simulink model "TCMSSystem"  (R2019b)
settings: configuration reference "ConfigSet_TCMSSystem_Reference" (kept outside this file)
model workspace (MAT data in the model file):
  Prm_TCMSSystem = Simulink.Parameter
  Prm_TCMSSystem.Value.LoadCompensationMasses = [21000 33350]
  Prm_TCMSSystem.Value.LoadCompensationPressures = [165000 440000]
  Prm_TCMSSystem.Value.TractionAccelerationTargets = [0 1.36]
  Prm_TCMSSystem.Value.BrakingDecelerationTargets = [0 1.1]
  Prm_TCMSSystem.Value.TractionBrakingDemands = [0 100]
  Prm_TCMSSystem.Value.AW3TractionAccelerationTargets = [0 1.08]
  Prm_TCMSSystem.Value.AW3BrakingDecelerationTargets = [0 0.8]
  Prm_TCMSSystem.DataType = 'Bus: BD_TCMSSystem_Prm'
  Prm_TCMSSystem.Dimensions = [1 1]
  SampleTime = 0.05
undefined symbols (not defined in the file): ADDIntervention, AK1Status, AK2Status, AKContactorStatus, AllDoorsClosed, AllLeftDoorsClosed, AllRightDoorsClosed, APS1Fault, APS1Isolated, APS1OutputVoltage, APS1Status, APS2Fault, APS2Isolated, APS2OutputVoltage, APS2Status, APSKAKContactor, ASCOEnd1, ASCOEnd2, ATBMode, ATCBypassMode, ATCStatusNotOK, ATOMode, ATPLowSpeedCutoutStatus, ATPMode, AuxCompressor, BatteryCurrent, BatteryIsolationContactor, BatteryTemperature, BatteryVoltage, BCG1Fault, BCG1Isolated, BCG1IsolationFailed, BCG1OutputCurrent, BCG1Status, BCG2Fault, BCG2Isolated, BCG2OutputCurrent, BCG2Status, BCGOutputVoltage, BECU1AxleLockedWheelSet1, BECU2AxleLockedWheelSet2, BECUFaulty, BECUMajorFault, BECUMinorFault, BECUStatus, BIC1Inside, BIC1Outside, BIC2Inside, BIC2Outside, Bogie, Bogie1WSPStatus, Bogie2WSPStatus, BogieFaulty, BogieIsolationStatus, BogieSupportedMass, BrakeCylinderPressureGauge, BrakeLoopCBTripped, BrakeLoopOpenTL, BrakeTrainLineStatus, BrakingDemand ... (+215)
libraries: TimersLib x257, simulink x137, LatchesLib x42, VectorOperationsLib x15, TestBenchLib x12, MathOperationsLib x2, FiltersLib x1
(part 1 of 16)
settings Model: ParameterArgumentNames=Prm_TCMSSystem  Creator=cdyer  LastModifiedBy=hinganes
settings ConfigSetRef: SourceName=ConfigSet_TCMSSystem_Reference  SourceLocation=Base Workspace

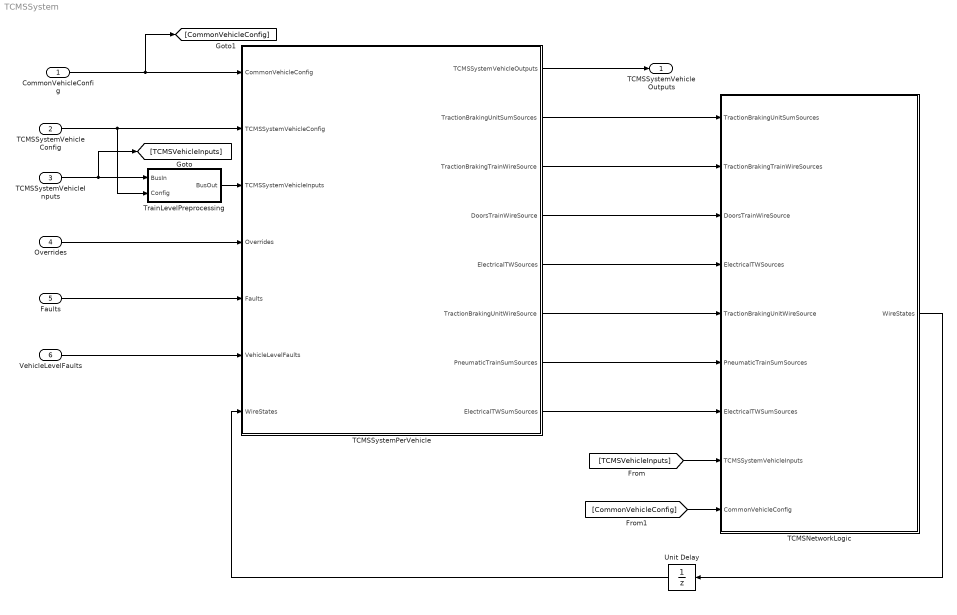
== system TCMSSystem ==
  CommonVehicleConfig : Inport  OutDataTypeStr=Bus: BD_CommonTrain_Cfg_Vehicle  PortDimensions=MaxVehicles  SampleTime=SampleTime  BusOutputAsStruct=on
  TCMSSystemVehicleConfig : Inport  Port=2  OutDataTypeStr=Bus: BD_TCMSSystem_Cfg_Vehicle  PortDimensions=MaxVehicles  SampleTime=SampleTime  BusOutputAsStruct=on
  TCMSSystemVehicleInputs : Inport  Port=3  OutDataTypeStr=Bus: BD_TCMSSystem_In_Vehicle  PortDimensions=MaxVehicles  SampleTime=SampleTime  BusOutputAsStruct=on
  Overrides : Inport  Port=4  OutDataTypeStr=Bus: BD_TCMSSystem_In_Vehicle_Overrides  PortDimensions=MaxVehicles  SampleTime=SampleTime  BusOutputAsStruct=on
  Faults : Inport  Port=5  OutDataTypeStr=Bus: BD_TCMSSystem_In_Vehicle_Faults  PortDimensions=MaxVehicles  SampleTime=SampleTime  BusOutputAsStruct=on
  VehicleLevelFaults : Inport  Port=6  OutDataTypeStr=Bus: BD_SimIntegration_Faults_Vehicle  PortDimensions=MaxVehicles  SampleTime=SampleTime  BusOutputAsStruct=on
  TCMSNetworkLogic : Subsystem  TreatAsAtomicUnit=on  SystemSampleTime=SampleTime
  TCMSSystemPerVehicle : Subsystem
  TrainLevelPreprocessing : Subsystem
  Unit Delay : UnitDelay  SampleTime=-1  HasFrameUpgradeWarning=on
  TCMSSystemVehicleOutputs : Outport  OutDataTypeStr=Bus: BD_TCMSSystem_Out_Vehicle  BusOutputAsStruct=on
  wires:
  CommonVehicleConfig/1 -> [CommonVehicleConfig], TCMSSystemPerVehicle/1(CommonVehicleConfig)
  TCMSSystemPerVehicle/1(TCMSSystemVehicleOutputs) -> TCMSSystemVehicleOutputs/1
  TCMSSystemVehicleConfig/1 -> TrainLevelPreprocessing/2(Config), TCMSSystemPerVehicle/2(TCMSSystemVehicleConfig)
  Overrides/1 -> TCMSSystemPerVehicle/4(Overrides)
  Faults/1 -> TCMSSystemPerVehicle/5(Faults)
  TCMSSystemPerVehicle/2(TractionBrakingUnitSumSources) -> TCMSNetworkLogic/1(TractionBrakingUnitSumSources)
  [TCMSVehicleInputs] -> TCMSNetworkLogic/8(TCMSSystemVehicleInputs)
  TCMSNetworkLogic/1(WireStates) -> Unit Delay/1
  Unit Delay/1 -> TCMSSystemPerVehicle/7(WireStates)
  TCMSSystemPerVehicle/3(TractionBrakingTrainWireSource) -> TCMSNetworkLogic/2(TractionBrakingTrainWireSources)
  TCMSSystemPerVehicle/4(DoorsTrainWireSource) -> TCMSNetworkLogic/3(DoorsTrainWireSource)
  TCMSSystemPerVehicle/5(ElectricalTWSources) -> TCMSNetworkLogic/4(ElectricalTWSources)
  [CommonVehicleConfig] -> TCMSNetworkLogic/9(CommonVehicleConfig)
  TCMSSystemPerVehicle/6(TractionBrakingUnitWireSource) -> TCMSNetworkLogic/5(TractionBrakingUnitWireSource)
  TCMSSystemPerVehicle/7(PneumaticTrainSumSources) -> TCMSNetworkLogic/6(PneumaticTrainSumSources)
  VehicleLevelFaults/1 -> TCMSSystemPerVehicle/6(VehicleLevelFaults)
  TCMSSystemPerVehicle/8(ElectricalTWSumSources) -> TCMSNetworkLogic/7(ElectricalTWSumSources)
  TCMSSystemVehicleInputs/1 -> [TCMSVehicleInputs], TrainLevelPreprocessing/1(BusIn)
  TrainLevelPreprocessing/1(BusOut) -> TCMSSystemPerVehicle/3(TCMSSystemVehicleInputs)

== system TCMSSystem/TCMSNetworkLogic ==
  TractionBrakingUnitSumSources : Inport  OutDataTypeStr=Bus: BD_TCMSSystem_Wires_TBUnitSum
  TractionBrakingTrainWireSources : Inport  Port=2  OutDataTypeStr=Bus: BD_TCMSSystem_Wires_TBTrainWire
  DoorsTrainWireSource : Inport  Port=3
  ElectricalTWSources : Inport  Port=4
  TractionBrakingUnitWireSource : Inport  Port=5
  PneumaticTrainSumSources : Inport  Port=6
  ElectricalTWSumSources : Inport  Port=7
  TCMSSystemVehicleInputs : Inport  Port=8  OutDataTypeStr=Bus: BD_TCMSSystem_In_Vehicle  PortDimensions=MaxVehicles  SampleTime=SampleTime  BusOutputAsStruct=on
  CommonVehicleConfig : Inport  Port=9
  ExtractConnections : Subsystem
  Goto Tag Visibility : GotoTagVisibility  GotoTag=Orientation
  Goto Tag Visibility1 : GotoTagVisibility  GotoTag=TrainConnection
  OrientationWiresLogic : Subsystem
  Terminator : Terminator
  TrainSumBus : VectorOperationsLib/TrainSumBus  OutDataTypeStr=Bus: BD_TCMSSystem_Wires_TBUnitSum
      settings: SourceProductName=Sydac Utilities
  TrainSumBus1 : VectorOperationsLib/TrainSumBus  OutDataTypeStr=Bus: BD_TCMSSystem_Wires_TBTrainWire
      settings: SourceProductName=Sydac Utilities
  TrainSumBus2 : VectorOperationsLib/TrainSumBus  OutDataTypeStr=Bus: BD_TCMSSystem_Wires_PneumaticTrainSum
      settings: SourceProductName=Sydac Utilities
  TrainSumBus3 : VectorOperationsLib/TrainSumBus  OutDataTypeStr=Bus: BD_TCMSSystem_Wires_ElectricalTrainSum
      settings: SourceProductName=Sydac Utilities
  TrainWiresBus : VectorOperationsLib/TrainWiresBus  OutDataTypeStr=Bus: BD_TCMSSystem_Wires_ElectricalTrainWire
      settings: SourceProductName=Sydac Utilities
  TrainWiresBus1 : VectorOperationsLib/TrainWiresBus  OutDataTypeStr=Bus: BD_TCMSSystem_Wires_TBUnitWire
      settings: SourceProductName=Sydac Utilities
  WireStatesRepack : Subsystem
  WireStates : Outport  OutDataTypeStr=Bus: BD_TCMSSystem_Wires
  tag scope: Orientation=scoped, TrainConnection=scoped
  wires:
  TractionBrakingUnitSumSources/1 -> TrainSumBus/1
  [UnitConnection] -> TrainSumBus/2
  TrainSumBus/1 -> WireStatesRepack/1(TractionBrakingUnitSumWireStates)
  TCMSSystemVehicleInputs/1 -> ExtractConnections/1(TCMSSystemVehicleInputs)
  ExtractConnections/1(UnitConnection) -> [UnitConnection]
  ExtractConnections/2(TrainConnection) -> [TrainConnection]
  [TrainConnection] -> TrainSumBus1/2
  TractionBrakingTrainWireSources/1 -> TrainSumBus1/1
  TrainSumBus1/1 -> WireStatesRepack/2(TractionBrakingTrainWireStates)
  WireStatesRepack/1(WireStates) -> WireStates/1
  ElectricalTWSources/1 -> TrainWiresBus/1
  [TrainConnection] -> TrainWiresBus/2
  TrainWiresBus/1 -> WireStatesRepack/4(ElectricalTrainWiresStates)
  CommonVehicleConfig/1 -> ExtractConnections/2(CommonVehicleConfig)
  ExtractConnections/3(Orientation) -> [Orientation]
  OrientationWiresLogic/1(WireStates) -> WireStatesRepack/3(DoorsTrainWiresStates)
  TractionBrakingUnitWireSource/1 -> TrainWiresBus1/1
  [UnitConnection] -> TrainWiresBus1/2
  TrainWiresBus1/1 -> WireStatesRepack/5(TractionBrakingUnitWire)
  TrainSumBus2/1 -> WireStatesRepack/6(PneumaticTrainSumSourcesWiresStates)
  PneumaticTrainSumSources/1 -> TrainSumBus2/1
  [TrainConnection] -> TrainSumBus2/2
  ElectricalTWSumSources/1 -> TrainSumBus3/1
  [TrainConnection] -> TrainSumBus3/2
  TrainSumBus3/1 -> WireStatesRepack/7(ElectricalTWSumSourcesWiresStates)
  [Orientation] -> Terminator/1
  DoorsTrainWireSource/1 -> OrientationWiresLogic/1(WireSources)

== system TCMSSystem/TCMSSystemPerVehicle ==
  CommonVehicleConfig : Inport  Partition=on  PartitionDimension=1  PartitionWidth=1  PartitionOffset=0
  TCMSSystemVehicleConfig : Inport  Port=2  Partition=on  PartitionDimension=1  PartitionWidth=1  PartitionOffset=0
  TCMSSystemVehicleInputs : Inport  Port=3  Partition=on  PartitionDimension=1  PartitionWidth=1  PartitionOffset=0
  Overrides : Inport  Port=4  Partition=on  PartitionDimension=1  PartitionWidth=1  PartitionOffset=0
  Faults : Inport  Port=5  Partition=on  PartitionDimension=1  PartitionWidth=1  PartitionOffset=0
  VehicleLevelFaults : Inport  Port=6  Partition=on  PartitionDimension=1  PartitionWidth=1  PartitionOffset=0
  WireStates : Inport  Port=7  Partition=on  PartitionDimension=1  PartitionWidth=1  PartitionOffset=0
  AND : Logic  AllPortsSameDT=off  OutDataTypeStr=boolean
  Bus Selector1 : BusSelector  OutputSignals=Enabled
  Bus Selector2 : BusSelector  OutputSignals=ElectricalSignals.TCMSPowerAvailable,ElectricalSignals.LimpHomeMode
  Bus Selector3 : BusSelector  OutputSignals=TCMSFailure
  Data Type Conversion : DataTypeConversion  OutDataTypeStr=uint32
  Data Type Conversion1 : DataTypeConversion  OutDataTypeStr=uint32
  Data Type Conversion2 : DataTypeConversion  OutDataTypeStr=uint32
  DisabledTCMSVehicle : Subsystem
  EnabledTCMSVehicle : Subsystem
  For Each : ForEach  DisableCoverage=on
  If : If  NumInputs=3  IfExpression=u1 > 0 & u2 ==0 & u3 == 1  ElseIfExpressions=u2 == 1
  LimpHomeTCMSVehicle : Subsystem
  Merge1 : Merge
  Merge3 : Merge
  Merge4 : Merge  Inputs=3
  Merge5 : Merge
  NOT : Logic  Operator=NOT  AllPortsSameDT=off  OutDataTypeStr=boolean
  Unit Delay : UnitDelay  SampleTime=-1  HasFrameUpgradeWarning=on
  TCMSSystemVehicleOutputs : Outport  ConcatenationDimension=1
  TractionBrakingUnitSumSources : Outport  Port=2  ConcatenationDimension=1
  TractionBrakingTrainWireSource : Outport  Port=3  ConcatenationDimension=1
  DoorsTrainWireSource : Outport  Port=4  ConcatenationDimension=1
  ElectricalTWSources : Outport  Port=5  ConcatenationDimension=1
  TractionBrakingUnitWireSource : Outport  Port=6  ConcatenationDimension=1
  PneumaticTrainSumSources : Outport  Port=7  ConcatenationDimension=1
  ElectricalTWSumSources : Outport  Port=8  ConcatenationDimension=1
  wires:
  CommonVehicleConfig/1 -> Bus Selector1/1, EnabledTCMSVehicle/1(CommonVehicleConfig)
  TCMSSystemVehicleConfig/1 -> DisabledTCMSVehicle/1(TCMSSystemVehicleConfig), LimpHomeTCMSVehicle/1(TCMSSystemVehicleConfig), EnabledTCMSVehicle/2(TCMSSystemVehicleConfig)
  Overrides/1 -> EnabledTCMSVehicle/4(Overrides)
  Faults/1 -> Bus Selector3/1, EnabledTCMSVehicle/5(TCMSFaults)
  Bus Selector2/1 -> AND/2  "<TCMSPowerAvailable>"
  Bus Selector1/1 -> AND/1  "<Enabled>"
  LimpHomeTCMSVehicle/3(NoTCMSSystemVehicleOutputs) -> Merge4/1
  If/2 -> LimpHomeTCMSVehicle/Action  "LimpHome"
  AND/1 -> Data Type Conversion/1
  If/1 -> EnabledTCMSVehicle/Action  "HealthyTCMS"
  Data Type Conversion/1 -> If/1
  EnabledTCMSVehicle/1(TractionBrakingUnitSumSources) -> Merge1/1
  WireStates/1 -> LimpHomeTCMSVehicle/3(WireStates), EnabledTCMSVehicle/6(WireStates)
  EnabledTCMSVehicle/2(TractionBrakingTrainWireSource) -> Merge5/1
  EnabledTCMSVehicle/4(DoorsTrainWireSource) -> DoorsTrainWireSource/1
  EnabledTCMSVehicle/3(ElectricalTWSources) -> ElectricalTWSources/1
  TCMSSystemVehicleInputs/1 -> Bus Selector2/1, LimpHomeTCMSVehicle/2(TCMSSystemInputs), EnabledTCMSVehicle/3(TCMSSystemInputs)
  Merge5/1 -> TractionBrakingTrainWireSource/1
  Merge1/1 -> TractionBrakingUnitSumSources/1
  LimpHomeTCMSVehicle/1(TractionBrakingUnitSumSources) -> Merge1/2
  LimpHomeTCMSVehicle/2(TractionBrakingTrainWireSource) -> Merge5/2
  Merge3/1 -> TractionBrakingUnitWireSource/1
  EnabledTCMSVehicle/6(TractionBrakingUnitWireSources) -> Merge3/1
  LimpHomeTCMSVehicle/4(TractionBrakingUnitWireSources) -> Merge3/2
  Bus Selector2/2 -> Data Type Conversion1/1  "<LimpHomeMode>"
  Data Type Conversion1/1 -> If/2
  If/3 -> DisabledTCMSVehicle/Action  "TCMSFailed"
  DisabledTCMSVehicle/1(NoTCMSSystemVehicleOutputs) -> Merge4/3
  EnabledTCMSVehicle/7(PneumaticTrainSumSources) -> PneumaticTrainSumSources/1
  VehicleLevelFaults/1 -> EnabledTCMSVehicle/7(VehicleLevelFaults)
  EnabledTCMSVehicle/8(ElectricalTWSumSources) -> ElectricalTWSumSources/1
  [TCMSSystemVehicleOutputs] -> Unit Delay/1
  Bus Selector3/1 -> NOT/1  "<TCMSFailure>"
  Unit Delay/1 -> LimpHomeTCMSVehicle/4(TCMSSystemVehicleOutputs)
  EnabledTCMSVehicle/5(TCMSSystemVehicleOutputs) -> Merge4/2
  Merge4/1 -> [TCMSSystemVehicleOutputs], TCMSSystemVehicleOutputs/1
  NOT/1 -> Data Type Conversion2/1
  Data Type Conversion2/1 -> If/3

== system TCMSSystem/TrainLevelPreprocessing ==
  BusIn : Inport
  Config : Inport  Port=2
  AND1 : Logic  AllPortsSameDT=off  OutDataTypeStr=boolean
  AND2 : Logic  AllPortsSameDT=off  OutDataTypeStr=boolean
  Add : Sum  Inputs=1
  Add1 : Sum  Inputs=1
  Add2 : Sum  Inputs=2
  Add3 : Sum  Inputs=1
  Assignment : Subsystem
  Data Type Conversion : DataTypeConversion  OutDataTypeStr=double
  Data Type Conversion1 : DataTypeConversion  OutDataTypeStr=double
  Data Type Conversion2 : DataTypeConversion  OutDataTypeStr=double
  Detect Decrease1 : simulink/Logic and Bit Operations/Detect Decrease  vinit=0.0  OutDataTypeStr=boolean
  Detect Increase : simulink/Logic and Bit Operations/Detect Increase  vinit=0.0  OutDataTypeStr=boolean
  EdgeCounter : LatchesLib/EdgeCounter
      settings: SourceProductName=Latches
  Logical Operator : Logic  Operator=OR  Inputs=1  AllPortsSameDT=off  OutDataTypeStr=boolean
  Logical Operator1 : Logic  Operator=NOT  Inputs=1  AllPortsSameDT=off  OutDataTypeStr=boolean
  Logical Operator2 : Logic  Operator=OR  Inputs=1  AllPortsSameDT=off  OutDataTypeStr=boolean
  Logical Operator3 : Logic  Operator=OR  Inputs=1  AllPortsSameDT=off  OutDataTypeStr=boolean
  Subsystem : Subsystem
  Subsystem1 : Subsystem
  Subsystem2 : Subsystem
  Subsystem3 : Subsystem
  BusOut : Outport
  wires:
  BusIn/1 -> Subsystem2/1(In1), Subsystem1/1(In1), Subsystem/1(In1), Assignment/1(In1)
  Detect Increase/1 -> EdgeCounter/1
  EdgeCounter/1 -> Assignment/2(VehiclesPassedNS)
  Subsystem/1(<NeutralSection>) -> Logical Operator/1, AND1/1
  Assignment/1(Out1) -> BusOut/1
  Logical Operator/1 -> Logical Operator1/1, Detect Increase/1
  Config/1 -> Subsystem2/2(In2), Subsystem3/1(In1)
  Subsystem3/1(<Enabled>) -> AND1/2
  AND1/1 -> Logical Operator2/1  "LastCarPassedNS"
  Logical Operator2/1 -> Detect Decrease1/1
  Detect Decrease1/1 -> AND2/2  "EndOfCar"
  AND2/1 -> EdgeCounter/2  "LastCarPassedNS"
  Logical Operator1/1 -> AND2/1
  Subsystem1/1(<ADDFault>) -> Logical Operator3/1
  Logical Operator3/1 -> Assignment/3(ADDInter)
  Subsystem2/1(APS1Unhealthy) -> Data Type Conversion/1
  Subsystem2/2(APS2Unhealthy) -> Data Type Conversion1/1
  Add/1 -> Add2/1
  Add1/1 -> Add2/2
  Add2/1 -> Assignment/4(NoOfAPSFaulty)
  Data Type Conversion/1 -> Add/1
  Data Type Conversion1/1 -> Add1/1
  Subsystem2/3(EPIC) -> Data Type Conversion2/1
  Add3/1 -> Assignment/5(NoOfEPICCutout)
  Data Type Conversion2/1 -> Add3/1

== system TCMSSystem/TCMSNetworkLogic/ExtractConnections ==
  TCMSSystemVehicleInputs : Inport  Partition=on  PartitionDimension=1  PartitionWidth=1  PartitionOffset=0
  CommonVehicleConfig : Inport  Port=2  Partition=on  PartitionDimension=1  PartitionWidth=1  PartitionOffset=0
  Bus Selector : BusSelector  OutputSignals=CouplingSystem.UnitConnection,CouplingSystem.TrainConnection
  Bus Selector2 : BusSelector  OutputSignals=Orientation
  For Each : ForEach  DisableCoverage=on
  UnitConnection : Outport  ConcatenationDimension=1
  TrainConnection : Outport  Port=2  ConcatenationDimension=1
  Orientation : Outport  Port=3  ConcatenationDimension=1
  wires:
  Bus Selector/1 -> UnitConnection/1  "<UnitConnection>"
  TCMSSystemVehicleInputs/1 -> Bus Selector/1
  Bus Selector/2 -> TrainConnection/1  "<TrainConnection>"
  Bus Selector2/1 -> Orientation/1  "<Orientation>"
  CommonVehicleConfig/1 -> Bus Selector2/1

== system TCMSSystem/TCMSNetworkLogic/OrientationWiresLogic ==
  WireSources : Inport
  PartitionWireSources : Subsystem  TreatAsAtomicUnit=on
  Train Wire Pair Swap1 : VectorOperationsLib/Train Wire Pair Swap
      settings: SourceProductName=Sydac Utilities
  Train Wire Pair Swap3 : VectorOperationsLib/Train Wire Pair Swap
      settings: SourceProductName=Sydac Utilities
  WiresStatesRepack : Subsystem  TreatAsAtomicUnit=on
  WireStates : Outport
  wires:
  PartitionWireSources/4(RDCReq) -> Train Wire Pair Swap1/2
  Train Wire Pair Swap3/1 -> WiresStatesRepack/1(LDOReq)  "TW21201"
  PartitionWireSources/2(RDOReq) -> Train Wire Pair Swap3/2
  Train Wire Pair Swap1/2 -> WiresStatesRepack/4(RDCReq)  "TW81106"
  WireSources/1 -> PartitionWireSources/1(In1)
  Train Wire Pair Swap3/2 -> WiresStatesRepack/2(RDOReq)  "TW21202"
  PartitionWireSources/3(LDCReq) -> Train Wire Pair Swap1/1
  Train Wire Pair Swap1/1 -> WiresStatesRepack/3(LDCReq)  "TW81105"
  PartitionWireSources/1(LDOReq) -> Train Wire Pair Swap3/1
  WiresStatesRepack/1(Out1) -> WireStates/1
  [TrainConnection] -> Train Wire Pair Swap3/4
  [Orientation] -> Train Wire Pair Swap3/3
  [Orientation] -> Train Wire Pair Swap1/3
  [TrainConnection] -> Train Wire Pair Swap1/4

== system TCMSSystem/TCMSNetworkLogic/WireStatesRepack ==
  TractionBrakingUnitSumWireStates : Inport  Partition=on  PartitionDimension=1  PartitionWidth=1  PartitionOffset=0
  TractionBrakingTrainWireStates : Inport  Port=2  Partition=on  PartitionDimension=1  PartitionWidth=1  PartitionOffset=0
  DoorsTrainWiresStates : Inport  Port=3  Partition=on  PartitionDimension=1  PartitionWidth=1  PartitionOffset=0
  ElectricalTrainWiresStates : Inport  Port=4  Partition=on  PartitionDimension=1  PartitionWidth=1  PartitionOffset=0
  TractionBrakingUnitWire : Inport  Port=5  Partition=on  PartitionDimension=1  PartitionWidth=1  PartitionOffset=0
  PneumaticTrainSumSourcesWiresStates : Inport  Port=6  Partition=on  PartitionDimension=1  PartitionWidth=1  PartitionOffset=0
  ElectricalTWSumSourcesWiresStates : Inport  Port=7  Partition=on  PartitionDimension=1  PartitionWidth=1  PartitionOffset=0
  Bus Creator : BusCreator  Inputs=7  OutDataTypeStr=Bus: BD_TCMSSystem_Wires  NonVirtualBus=on
  For Each : ForEach  DisableCoverage=on
  WireStates : Outport  ConcatenationDimension=1
  wires:
  TractionBrakingUnitSumWireStates/1 -> Bus Creator/1  "TractionBrakingUnitSum"
  TractionBrakingTrainWireStates/1 -> Bus Creator/2  "TractionBrakingTrainWire"
  Bus Creator/1 -> WireStates/1
  DoorsTrainWiresStates/1 -> Bus Creator/3  "DoorsTrainWire"
  ElectricalTrainWiresStates/1 -> Bus Creator/4  "ElectricalTrainWire"
  TractionBrakingUnitWire/1 -> Bus Creator/5  "TractionBrakingUnitWire"
  PneumaticTrainSumSourcesWiresStates/1 -> Bus Creator/6  "PneumaticTrainSum"
  ElectricalTWSumSourcesWiresStates/1 -> Bus Creator/7  "ElectricalTrainSum"

== system TCMSSystem/TCMSSystemPerVehicle/DisabledTCMSVehicle ==
  TCMSSystemVehicleConfig : Inport
  Action Port : ActionPort  ActionPortLabel=else
  Bus Assignment1 : BusAssignment  AssignedSignals=Display.ElectricalSystem.HMIPower
  Bus Selector : BusSelector  OutputSignals=HMIPower
  CabUnitDisplay : Subsystem
  Constant3 : Constant  Value=0  OutDataTypeStr=Bus: BD_TCMSSystem_Out_Vehicle
  NoTCMSSystemVehicleOutputs : Outport  OutDataTypeStr=Bus: BD_TCMSSystem_Out_Vehicle
  wires:
  CabUnitDisplay/1(CabUnitDisplay) -> Bus Selector/1  "CabUnitDisplay"
  Bus Selector/1 -> Bus Assignment1/2  "<HMIPower>"
  Constant3/1 -> Bus Assignment1/1
  Bus Assignment1/1 -> NoTCMSSystemVehicleOutputs/1
  TCMSSystemVehicleConfig/1 -> CabUnitDisplay/1(TCMSConfig)

== system TCMSSystem/TCMSSystemPerVehicle/EnabledTCMSVehicle ==
  CommonVehicleConfig : Inport
  TCMSSystemVehicleConfig : Inport  Port=2
  TCMSSystemInputs : Inport  Port=3
  Overrides : Inport  Port=4
  TCMSFaults : Inport  Port=5
  WireStates : Inport  Port=6
  VehicleLevelFaults : Inport  Port=7
  Action Port : ActionPort  ActionPortLabel=if(u1 > 0 & u2 ==0 & u3 == 1)
  OutputsPacking : Subsystem
  TCMSDoors : Subsystem
  TCMSElectrical : Subsystem
  TCMSPantograph : Subsystem
  TCMSPneumatics : Subsystem
  TCMSStatus : Subsystem
  TCMSTractionBraking : Subsystem
  Terminator2 : Terminator
  TractionBrakingUnitSumSources : Outport  OutDataTypeStr=Bus: BD_TCMSSystem_Wires_TBUnitSum
  TractionBrakingTrainWireSource : Outport  Port=2  OutDataTypeStr=Bus: BD_TCMSSystem_Wires_TBTrainWire  LockScale=on
  ElectricalTWSources : Outport  Port=3
  DoorsTrainWireSource : Outport  Port=4  OutDataTypeStr=Bus: BD_TCMSSystem_Wires_DoorsTrainWire  LockScale=on
  TCMSSystemVehicleOutputs : Outport  Port=5  OutDataTypeStr=Bus: BD_TCMSSystem_Out_Vehicle
  TractionBrakingUnitWireSources : Outport  Port=6  OutDataTypeStr=Bus: BD_TCMSSystem_Wires_TBUnitWire
  PneumaticTrainSumSources : Outport  Port=7  OutDataTypeStr=Bus: BD_TCMSSystem_Wires_PneumaticTrainSum
  ElectricalTWSumSources : Outport  Port=8
  wires:
  OutputsPacking/1(TCMSSystemVehicleOutputs) -> TCMSSystemVehicleOutputs/1
  TCMSFaults/1 -> OutputsPacking/7(TCMSFaults), TCMSTractionBraking/4(Faults), TCMSElectrical/4(TCMSFaults), TCMSStatus/3(TCMSFaults)
  Overrides/1 -> Terminator2/1
  TCMSTractionBraking/1(TractionBrakingOut) -> TCMSPneumatics/5(TractionBrakingFB), OutputsPacking/4(TractionBrakingOut)
  TCMSPantograph/1(PantographOut) -> OutputsPacking/2(PantographOut)
  CommonVehicleConfig/1 -> TCMSElectrical/6(CommonVehicleConfig), TCMSDoors/1(CommonVehicleConfig)
  TCMSDoors/1(DoorsOut) -> OutputsPacking/1(DoorsOut)
  TCMSTractionBraking/2(TractionBrakingUnitSumSources) -> TractionBrakingUnitSumSources/1
  WireStates/1 -> TCMSElectrical/3(WireStates), TCMSPneumatics/4(WireStates), TCMSDoors/4(WireStates), TCMSTractionBraking/3(WireStates)
  TCMSTractionBraking/3(TractionBrakingTrainWireSource) -> TractionBrakingTrainWireSource/1
  TCMSSystemVehicleConfig/1 -> TCMSStatus/1(TCMSSystemVehicleConfig), TCMSElectrical/1(TCMSSystemVehicleConfig), TCMSTractionBraking/1(TCMSSystemVehicleConfig), TCMSPneumatics/1(TCMSSystemVehicleConfig), TCMSPantograph/1(TCMSSystemVehicleConfig), TCMSDoors/2(TCMSSystemVehicleConfig)
  TCMSPneumatics/1(PneumaticsOut) -> OutputsPacking/3(PneumaticsOut)
  TCMSElectrical/1(ElectricalOut) -> OutputsPacking/5(ElectricalOut)
  TCMSDoors/2(DoorsTrainWireSources) -> DoorsTrainWireSource/1
  TCMSSystemInputs/1 -> OutputsPacking/9(TCMSInputs), TCMSStatus/2(TCMSSystemInputs), TCMSElectrical/2(TCMSSystemInputs), TCMSTractionBraking/2(TCMSSystemInputs), TCMSPneumatics/2(TCMSSystemInputs), TCMSPantograph/2(TCMSSystemInputs), TCMSDoors/3(TCMSSystemInputs)
  TCMSElectrical/2(ElectricalTWSources) -> ElectricalTWSources/1
  TCMSStatus/1(TCMSStatus) -> OutputsPacking/6(TCMSStatus)
  TCMSTractionBraking/4(TractionBrakingUnitWireSources) -> TractionBrakingUnitWireSources/1
  TCMSPneumatics/2(PneumaticTrainSumSources) -> PneumaticTrainSumSources/1
  VehicleLevelFaults/1 -> TCMSTractionBraking/5(VehicleFaults), TCMSPneumatics/3(VehicleFaults), TCMSElectrical/5(VehicleFaults), OutputsPacking/8(VehicleLevelFaults)
  TCMSElectrical/3(ElectricalTWSumSources) -> ElectricalTWSumSources/1

== system TCMSSystem/TCMSSystemPerVehicle/LimpHomeTCMSVehicle ==
  TCMSSystemVehicleConfig : Inport
  TCMSSystemInputs : Inport  Port=2
  WireStates : Inport  Port=3
  TCMSSystemVehicleOutputs : Inport  Port=4
  Action Port : ActionPort  ActionPortLabel=elseif(u2 == 1)
  Bus Assignment : BusAssignment  AssignedSignals=Control.TractionSBraking
  Bus Assignment1 : BusAssignment  AssignedSignals=Display.ElectricalSystem.HMIPower
  Bus Selector : BusSelector  OutputSignals=HMIPower
  CabUnitDisplay : Subsystem
  TCMSTractionBraking : Subsystem
  TractionBrakingUnitSumSources : Outport  OutDataTypeStr=Bus: BD_TCMSSystem_Wires_TBUnitSum
  TractionBrakingTrainWireSource : Outport  Port=2  OutDataTypeStr=Bus: BD_TCMSSystem_Wires_TBTrainWire  LockScale=on
  NoTCMSSystemVehicleOutputs : Outport  Port=3  OutDataTypeStr=Bus: BD_TCMSSystem_Out_Vehicle
  TractionBrakingUnitWireSources : Outport  Port=4  OutDataTypeStr=Bus: BD_TCMSSystem_Wires_TBUnitWire  LockScale=on
  wires:
  TCMSSystemVehicleConfig/1 -> CabUnitDisplay/1(TCMSConfig), TCMSTractionBraking/1(TCMSSystemVehicleConfig)
  WireStates/1 -> TCMSTractionBraking/3(WireStates)
  Bus Assignment1/1 -> NoTCMSSystemVehicleOutputs/1
  TCMSSystemVehicleOutputs/1 -> Bus Assignment/1
  TCMSTractionBraking/3(TractionBrakingTrainWireSource) -> TractionBrakingTrainWireSource/1
  TCMSTractionBraking/2(TractionBrakingUnitSumSources) -> TractionBrakingUnitSumSources/1
  TCMSTractionBraking/1(TractionBrakingControls) -> Bus Assignment/2
  TCMSTractionBraking/4(TractionBrakingUnitWireSources) -> TractionBrakingUnitWireSources/1
  Bus Assignment/1 -> Bus Assignment1/1
  TCMSSystemInputs/1 -> CabUnitDisplay/2(ElectricalSignals), TCMSTractionBraking/2(TCMSSystemInputs)
  Bus Selector/1 -> Bus Assignment1/2  "<HMIPower>"
  CabUnitDisplay/1(CabUnitDisplay) -> Bus Selector/1  "CabUnitDisplay"

== system TCMSSystem/TrainLevelPreprocessing/Assignment ==
  In1 : Inport  Partition=on  PartitionDimension=1  PartitionWidth=1  PartitionOffset=0
  VehiclesPassedNS : Inport  Port=2  Partition=on  PartitionDimension=1  PartitionWidth=1  PartitionOffset=0
  ADDInter : Inport  Port=3
  NoOfAPSFaulty : Inport  Port=4
  NoOfEPICCutout : Inport  Port=5
  Bus Assignment : BusAssignment  AssignedSignals=Environment.VehiclesPassedNS,PantographSystem.BrakeLoopADDIntervention,ElectricalSignals.NoOfAPSFailed,ElectricalSignals.NoOfEPICCutout
  For Each : ForEach  DisableCoverage=on
  Out1 : Outport  ConcatenationDimension=1
  wires:
  VehiclesPassedNS/1 -> Bus Assignment/2
  In1/1 -> Bus Assignment/1
  Bus Assignment/1 -> Out1/1
  ADDInter/1 -> Bus Assignment/3
  NoOfAPSFaulty/1 -> Bus Assignment/4
  NoOfEPICCutout/1 -> Bus Assignment/5

== system TCMSSystem/TrainLevelPreprocessing/Subsystem ==
  In1 : Inport  Partition=on  PartitionDimension=1  PartitionWidth=1  PartitionOffset=0
  Bus Selector : BusSelector  OutputSignals=Environment.NeutralSection
  For Each : ForEach  DisableCoverage=on
  <NeutralSection> : Outport  ConcatenationDimension=1
  wires:
  In1/1 -> Bus Selector/1
  Bus Selector/1 -> <NeutralSection>/1  "<NeutralSection>"

== system TCMSSystem/TrainLevelPreprocessing/Subsystem1 ==
  In1 : Inport  Partition=on  PartitionDimension=1  PartitionWidth=1  PartitionOffset=0
  Bus Selector : BusSelector  OutputSignals=PantographSystem.PantoADDFaultMessage
  For Each : ForEach  DisableCoverage=on
  <ADDFault> : Outport  ConcatenationDimension=1
  wires:
  Bus Selector/1 -> <ADDFault>/1  "<PantoADDFaultMessage>"
  In1/1 -> Bus Selector/1

== system TCMSSystem/TrainLevelPreprocessing/Subsystem2 ==
  In1 : Inport  Partition=on  PartitionDimension=1  PartitionWidth=1  PartitionOffset=0
  In2 : Inport  Port=2  Partition=on  PartitionDimension=1  PartitionWidth=1  PartitionOffset=0
  Bus Selector : BusSelector  OutputSignals=ElectricalSignals.APS1Status,ElectricalSignals.APS2Status,InputControlStates.EPIC
  Bus Selector1 : BusSelector  OutputSignals=HasVCB
  Compare To Zero : simulink/Logic and Bit Operations/Compare To Zero  relop===  OutDataTypeStr=boolean
  Compare To Zero1 : simulink/Logic and Bit Operations/Compare To Zero  relop===  OutDataTypeStr=boolean
  For Each : ForEach  DisableCoverage=on
  Logical Operator : Logic  AllPortsSameDT=off  OutDataTypeStr=boolean
  Logical Operator1 : Logic  AllPortsSameDT=off  OutDataTypeStr=boolean
  Logical Operator4 : Logic  Operator=NOT  Inputs=1  AllPortsSameDT=off  OutDataTypeStr=boolean
  APS1Unhealthy : Outport  ConcatenationDimension=1
  APS2Unhealthy : Outport  Port=2  ConcatenationDimension=1
  EPIC : Outport  Port=3  ConcatenationDimension=1
  wires:
  In1/1 -> Bus Selector/1
  Bus Selector/1 -> Compare To Zero/1  "<APS1Status>"
  Bus Selector/2 -> Compare To Zero1/1  "<APS2Status>"
  Compare To Zero1/1 -> Logical Operator1/1
  Compare To Zero/1 -> Logical Operator/1
  Logical Operator/1 -> APS1Unhealthy/1
  Logical Operator1/1 -> APS2Unhealthy/1
  In2/1 -> Bus Selector1/1
  Bus Selector1/1 -> Logical Operator1/2, Logical Operator/2  "<HasVCB>"
  Bus Selector/3 -> Logical Operator4/1  "<EPIC>"
  Logical Operator4/1 -> EPIC/1

== system TCMSSystem/TrainLevelPreprocessing/Subsystem3 ==
  In1 : Inport  Partition=on  PartitionDimension=1  PartitionWidth=1  PartitionOffset=0
  Bus Selector : BusSelector  OutputSignals=IsLastVehicle
  For Each : ForEach  DisableCoverage=on
  <Enabled> : Outport  ConcatenationDimension=1
  wires:
  In1/1 -> Bus Selector/1
  Bus Selector/1 -> <Enabled>/1  "<IsLastVehicle>"

== system TCMSSystem/TCMSNetworkLogic/OrientationWiresLogic/PartitionWireSources ==
  In1 : Inport  Partition=on  PartitionDimension=1  PartitionWidth=1  PartitionOffset=0
  Bus Selector : BusSelector  OutputSignals=LeftDoorOpenRequest,RightDoorOpenRequest,LeftDoorCloseRequest,RightDoorCloseRequest
  For Each : ForEach  DisableCoverage=on
  LDOReq : Outport  ConcatenationDimension=1
  RDOReq : Outport  Port=2  ConcatenationDimension=1
  LDCReq : Outport  Port=3  ConcatenationDimension=1
  RDCReq : Outport  Port=4  ConcatenationDimension=1
  wires:
  Bus Selector/4 -> RDCReq/1  "<RightDoorCloseRequest>"
  Bus Selector/3 -> LDCReq/1  "<LeftDoorCloseRequest>"
  Bus Selector/2 -> RDOReq/1  "<RightDoorOpenRequest>"
  Bus Selector/1 -> LDOReq/1  "<LeftDoorOpenRequest>"
  In1/1 -> Bus Selector/1

== system TCMSSystem/TCMSNetworkLogic/OrientationWiresLogic/WiresStatesRepack ==
  LDOReq : Inport  Partition=on  PartitionDimension=1  PartitionWidth=1  PartitionOffset=0
  RDOReq : Inport  Port=2  Partition=on  PartitionDimension=1  PartitionWidth=1  PartitionOffset=0
  LDCReq : Inport  Port=3  Partition=on  PartitionDimension=1  PartitionWidth=1  PartitionOffset=0
  RDCReq : Inport  Port=4  Partition=on  PartitionDimension=1  PartitionWidth=1  PartitionOffset=0
  Bus Creator : BusCreator  Inputs=4  OutDataTypeStr=Bus: BD_TCMSSystem_Wires_DoorsTrainWire  NonVirtualBus=on
  For Each : ForEach  DisableCoverage=on
  Out1 : Outport  ConcatenationDimension=1
  wires:
  Bus Creator/1 -> Out1/1
  LDOReq/1 -> Bus Creator/1  "LeftDoorOpenRequest"
  RDOReq/1 -> Bus Creator/2  "RightDoorOpenRequest"
  LDCReq/1 -> Bus Creator/3  "LeftDoorCloseRequest"
  RDCReq/1 -> Bus Creator/4  "RightDoorCloseRequest"

== system TCMSSystem/TCMSSystemPerVehicle/DisabledTCMSVehicle/CabUnitDisplay ==
  TCMSConfig : Inport
  Bus Selector1 : BusSelector  OutputSignals=HasCab
  CabActiveUnitDisplay : Subsystem  TreatAsAtomicUnit=on
  Data Type Conversion : DataTypeConversion  OutDataTypeStr=uint32
  If : If  ShowElse=off
  CabUnitDisplay : Outport
  wires:
  TCMSConfig/1 -> Bus Selector1/1
  Bus Selector1/1 -> Data Type Conversion/1  "<HasCab>"
  Data Type Conversion/1 -> If/1
  If/1 -> CabActiveUnitDisplay/Action
  CabActiveUnitDisplay/1(Out1) -> CabUnitDisplay/1

== system TCMSSystem/TCMSSystemPerVehicle/EnabledTCMSVehicle/OutputsPacking ==
  Bus Element In6 : Inport  PortName=DoorsOut  Element=Control
  In Bus Element5 : Inport  PortName=DoorsOut  Element=Control
  Bus Element In7 : Inport  PortName=DoorsOut  Element=Display
  Bus Element In : Inport  Port=2  PortName=PantographOut  Element=Control
  Bus Element In1 : Inport  Port=2  PortName=PantographOut  Element=Display
  Bus Element In5 : Inport  Port=3  PortName=PneumaticsOut  Element=Display
  In Bus Element6 : Inport  Port=3  PortName=PneumaticsOut  Element=Control
  In Bus Element8 : Inport  Port=3  PortName=PneumaticsOut  Element=Control
  Bus Element In2 : Inport  Port=4  PortName=TractionBrakingOut  Element=Control
  Bus Element In8 : Inport  Port=4  PortName=TractionBrakingOut  Element=Control
  Bus Element In3 : Inport  Port=4  PortName=TractionBrakingOut  Element=Display
  Bus Element In4 : Inport  Port=5  PortName=ElectricalOut  Element=Display
  In Bus Element : Inport  Port=5  PortName=ElectricalOut  Element=Control
  In Bus Element4 : Inport  Port=5  PortName=ElectricalOut  Element=Control
  In Bus Element3 : Inport  Port=6  PortName=TCMSStatus  Element=Display
  In Bus Element2 : Inport  Port=7  PortName=TCMSFaults
  In Bus Element1 : Inport  Port=7  PortName=TCMSFaults  Element=TCMSDisplayHanged
  VehicleLevelFaults : Inport  Port=8
  In Bus Element7 : Inport  Port=9  PortName=TCMSInputs  Element=InputControlStates
  Bus Assignment : BusAssignment  AssignedSignals=Control,Display
  Constant3 : Constant  Value=0  OutDataTypeStr=Bus: BD_TCMSSystem_Out_Vehicle
  NOT : Logic  Operator=NOT  AllPortsSameDT=off  OutDataTypeStr=boolean
  TCMSControlOutputs : Subsystem
  TCMSDisplayOutputs : Subsystem
  Terminator : Terminator
  TCMSSystemVehicleOutputs : Outport  OutDataTypeStr=Bus: BD_TCMSSystem_Out_Vehicle
  wires:
  Bus Element In8/1 -> TCMSDisplayOutputs/11(TractionControl)
  In Bus Element5/1 -> TCMSDisplayOutputs/10(DoorsControl)
  Bus Element In/1 -> TCMSControlOutputs/1(PangraphOut)
  In Bus Element4/1 -> TCMSDisplayOutputs/9(ElectricalControls)
  Bus Assignment/1 -> TCMSSystemVehicleOutputs/1
  NOT/1 -> TCMSDisplayOutputs/Enable
  Bus Element In6/1 -> TCMSControlOutputs/3(DoorsOut)
  In Bus Element1/1 -> NOT/1
  VehicleLevelFaults/1 -> TCMSDisplayOutputs/8(VehicleLevelFaults)
  In Bus Element3/1 -> TCMSDisplayOutputs/7(TCMSSystem)
  In Bus Element/1 -> TCMSControlOutputs/4(ElectricalOut)
  TCMSControlOutputs/1(TCMSControlOut) -> Bus Assignment/2
  In Bus Element2/1 -> TCMSDisplayOutputs/6(TCMSFaults)
  Bus Element In7/1 -> TCMSDisplayOutputs/4(DoorsOut)
  Bus Element In4/1 -> TCMSDisplayOutputs/5(ElectricalOut)
  Bus Element In1/1 -> TCMSDisplayOutputs/1(PangraphOut)
  Bus Element In5/1 -> TCMSDisplayOutputs/3(PneumaticsOut)
  Bus Element In2/1 -> TCMSControlOutputs/2(TractionOut)
  Bus Element In3/1 -> TCMSDisplayOutputs/2(TractionBrakingOut)
  Constant3/1 -> Bus Assignment/1
  TCMSDisplayOutputs/1(TCMSControlDisplay) -> Bus Assignment/3
  In Bus Element6/1 -> TCMSControlOutputs/5(PneumaticOut)
  In Bus Element7/1 -> Terminator/1
  In Bus Element8/1 -> TCMSDisplayOutputs/12(PneumaticsControl)

== system TCMSSystem/TCMSSystemPerVehicle/EnabledTCMSVehicle/TCMSDoors ==
  CommonVehicleConfig : Inport
  TCMSSystemVehicleConfig : Inport  Port=2
  Bus Element In : Inport  Port=3  PortName=TCMSSystemInputs  Element=DisplayControl
  Bus Element In1 : Inport  Port=3  PortName=TCMSSystemInputs  Element=ElectricalSignals
  Bus Element In2 : Inport  Port=3  PortName=TCMSSystemInputs  Element=DoorSystem
  In Bus Element : Inport  Port=3  PortName=TCMSSystemInputs  Element=CBTC
  In Bus Element1 : Inport  Port=3  PortName=TCMSSystemInputs  Element=InputControlStates
  In Bus Element2 : Inport  Port=4  PortName=WireStates  Element=DoorsTrainWire
  Bus Creator : BusCreator  Inputs=2
  CabControlsExtract : Subsystem  TreatAsAtomicUnit=on
  DoorsControl : Subsystem
  DoorsDisplay : Subsystem
  DoorsOut : Outport
  DoorsTrainWireSources : Outport  Port=2
  wires:
  TCMSSystemVehicleConfig/1 -> CabControlsExtract/1(TCMSConfig), DoorsDisplay/2(TCMSSystemVehicleConfig)
  Bus Element In2/1 -> DoorsDisplay/4(DoorSystem)
  Bus Element In1/1 -> DoorsDisplay/3(ElectricalSignals), CabControlsExtract/2(ElectricalSignals), DoorsControl/2(ElectricalSignals)
  Bus Element In/1 -> DoorsControl/1(DisplayControl)
  DoorsDisplay/1(Display) -> Bus Creator/2
  DoorsControl/1(Control) -> Bus Creator/1
  Bus Creator/1 -> DoorsOut/1  "DoorsOut"
  In Bus Element/1 -> CabControlsExtract/3(CBTCSignals)
  CommonVehicleConfig/1 -> DoorsControl/4(In4), DoorsDisplay/1(CommonVehicleConfig)
  CabControlsExtract/1(DoorsTrainWireSource) -> DoorsTrainWireSources/1
  In Bus Element2/1 -> DoorsControl/3(DoorWireStates)
  In Bus Element1/1 -> DoorsDisplay/5(InputControlStates)

== system TCMSSystem/TCMSSystemPerVehicle/EnabledTCMSVehicle/TCMSElectrical ==
  TCMSSystemVehicleConfig : Inport
  In Bus Element2 : Inport  Port=2  PortName=TCMSSystemInputs  Element=InputControlStates
  In Bus Element3 : Inport  Port=2  PortName=TCMSSystemInputs  Element=ElectricalSignals
  In Bus Element1 : Inport  Port=2  PortName=TCMSSystemInputs  Element=CBTC
  In Bus Element : Inport  Port=2  PortName=TCMSSystemInputs  Element=Environment
  In Bus Element5 : Inport  Port=2  PortName=TCMSSystemInputs  Element=DoorSystem
  In Bus Element6 : Inport  Port=2  PortName=TCMSSystemInputs  Element=DisplayControl
  In Bus Element7 : Inport  Port=2  PortName=TCMSSystemInputs  Element=TractionSystem
  In Bus Element10 : Inport  Port=2  PortName=TCMSSystemInputs  Element=PantographSystem
  In Bus Element12 : Inport  Port=2  PortName=TCMSSystemInputs  Element=CouplingSystem
  In Bus Element13 : Inport  Port=2  PortName=TCMSSystemInputs  Element=PneumaticsSystem
  In Bus Element4 : Inport  Port=3  PortName=WireStates
  In Bus Element11 : Inport  Port=3  PortName=WireStates  Element=ElectricalTrainSum
  In Bus Element8 : Inport  Port=4  PortName=TCMSFaults
  In Bus Element9 : Inport  Port=5  PortName=VehicleFaults
  CommonVehicleConfig : Inport  Port=6
  Bus Creator : BusCreator  Inputs=2
  ElectricalControl : Subsystem
  ElectricalDisplay : Subsystem
  ElectricalOut : Outport
  ElectricalTWSources : Outport  Port=2
  ElectricalTWSumSources : Outport  Port=3
  wires:
  TCMSSystemVehicleConfig/1 -> ElectricalControl/4(TCMSSystemVehicleConfig), ElectricalDisplay/1(TCMSSystemVehicleConfig)
  ElectricalDisplay/1(Display) -> Bus Creator/2  "Display"
  ElectricalControl/3(Control) -> Bus Creator/1  "Control"
  Bus Creator/1 -> ElectricalOut/1
  In Bus Element4/1 -> ElectricalDisplay/10(WireStates), ElectricalControl/1(WireStates)
  In Bus Element2/1 -> ElectricalControl/8(InputControlStates), ElectricalDisplay/4(InputControlStates)
  In Bus Element3/1 -> ElectricalControl/3(ElectricalSignals), ElectricalDisplay/3(ElectricalSignals)
  In Bus Element1/1 -> ElectricalControl/2(CBTC), ElectricalDisplay/5(CBTC)
  ElectricalControl/1(ElectricalTWSources) -> ElectricalTWSources/1
  In Bus Element/1 -> ElectricalControl/5(Environment)
  In Bus Element5/1 -> ElectricalControl/6(DoorSystem)
  In Bus Element6/1 -> ElectricalControl/7(DisplayControl)
  ElectricalControl/2(ElectricalTWSumSources) -> ElectricalTWSumSources/1
  In Bus Element8/1 -> ElectricalControl/9(TCMSFaults)
  In Bus Element9/1 -> ElectricalControl/10(VehicleFaults), ElectricalDisplay/6(VehicleFaults)
  In Bus Element7/1 -> ElectricalControl/11(TractionOut), ElectricalDisplay/8(TractionFB)
  In Bus Element10/1 -> ElectricalDisplay/9(PantographSignals), ElectricalControl/12(PantographSignals)
  In Bus Element11/1 -> ElectricalControl/13(ElectricalTrainSum)
  In Bus Element12/1 -> ElectricalDisplay/7(CouplingSystem)
  CommonVehicleConfig/1 -> ElectricalDisplay/2(CommonVehicleConfig)
  In Bus Element13/1 -> ElectricalControl/14(PneumaticsSignals)

== system TCMSSystem/TCMSSystemPerVehicle/EnabledTCMSVehicle/TCMSPantograph ==
  TCMSSystemVehicleConfig : Inport
  Bus Element In : Inport  Port=2  PortName=TCMSSystemInputs  Element=DisplayControl
  Bus Element In1 : Inport  Port=2  PortName=TCMSSystemInputs  Element=ElectricalSignals
  Bus Element In2 : Inport  Port=2  PortName=TCMSSystemInputs  Element=PantographSystem
  Bus Creator : BusCreator  Inputs=2
  PantographControl : Subsystem
  PantographDisplay : Subsystem
  PantographOut : Outport
  wires:
  Bus Creator/1 -> PantographOut/1  "PantographOut"
  PantographControl/1(Control) -> Bus Creator/1
  PantographDisplay/1(Display) -> Bus Creator/2
  Bus Element In/1 -> PantographControl/1(DisplayControl)
  Bus Element In1/1 -> PantographDisplay/2(ElectricalSignals)
  Bus Element In2/1 -> PantographDisplay/3(PantographSystem)
  TCMSSystemVehicleConfig/1 -> PantographDisplay/1(TCMSSystemVehicleConfig)

== system TCMSSystem/TCMSSystemPerVehicle/EnabledTCMSVehicle/TCMSPneumatics ==
  TCMSSystemVehicleConfig : Inport
  Bus Element In1 : Inport  Port=2  PortName=TCMSSystemInputs  Element=ElectricalSignals
  Bus Element In2 : Inport  Port=2  PortName=TCMSSystemInputs  Element=PneumaticsSystem
  In Bus Element : Inport  Port=2  PortName=TCMSSystemInputs  Element=InputControlStates
  In Bus Element1 : Inport  Port=2  PortName=TCMSSystemInputs  Element=DynamicsSystem
  In Bus Element2 : Inport  Port=3  PortName=VehicleFaults
  WireStates : Inport  Port=4
  In Bus Element3 : Inport  Port=5  PortName=TractionBrakingFB  Element=Control
  Bus Creator : BusCreator  Inputs=2
  PneumaticControl : Subsystem
  PneumaticsDisplay : Subsystem
  PneumaticsOut : Outport
  PneumaticTrainSumSources : Outport  Port=2
  wires:
  TCMSSystemVehicleConfig/1 -> PneumaticsDisplay/1(TCMSSystemVehicleConfig)
  Bus Element In2/1 -> PneumaticsDisplay/3(PneumaticsSystem)
  Bus Element In1/1 -> PneumaticsDisplay/2(ElectricalSignals)
  PneumaticsDisplay/1(Display) -> Bus Creator/2
  Bus Creator/1 -> PneumaticsOut/1  "PneumaticsOut"
  In Bus Element/1 -> PneumaticControl/2(IOControl), PneumaticsDisplay/4(IOControl)
  PneumaticsDisplay/2(PneumaticTrainSumSources) -> PneumaticTrainSumSources/1
  In Bus Element2/1 -> PneumaticsDisplay/5(PneumaticFaults)
  PneumaticControl/1(Control) -> Bus Creator/1
  WireStates/1 -> PneumaticControl/1(WireStates)
  In Bus Element3/1 -> PneumaticsDisplay/6(TractionBrakingFB)
  In Bus Element1/1 -> PneumaticsDisplay/7(Dynamics)

== system TCMSSystem/TCMSSystemPerVehicle/EnabledTCMSVehicle/TCMSStatus ==
  TCMSSystemVehicleConfig : Inport
  In Bus Element2 : Inport  Port=2  PortName=TCMSSystemInputs  Element=DisplayControl
  In Bus Element1 : Inport  Port=2  PortName=TCMSSystemInputs  Element=ElectricalSignals
  TCMSFaults : Inport  Port=3
  Bus Creator : BusCreator  Inputs=1
  TCMSSystemDisplay : Subsystem
  TCMSStatus : Outport
  wires:
  Bus Creator/1 -> TCMSStatus/1  "TCMSStatus"
  TCMSSystemDisplay/1(Display) -> Bus Creator/1
  TCMSSystemVehicleConfig/1 -> TCMSSystemDisplay/1(TCMSSystemVehicleConfig)
  In Bus Element2/1 -> TCMSSystemDisplay/2(DisplayControl)
  TCMSFaults/1 -> TCMSSystemDisplay/3(TCMSFaults)
  In Bus Element1/1 -> TCMSSystemDisplay/4(ElectricalIn)

== system TCMSSystem/TCMSSystemPerVehicle/EnabledTCMSVehicle/TCMSTractionBraking ==
  TCMSSystemVehicleConfig : Inport
  Bus Element In : Inport  Port=2  PortName=TCMSSystemInputs  Element=DisplayControl
  Bus Element In1 : Inport  Port=2  PortName=TCMSSystemInputs  Element=ElectricalSignals
  Bus Element In2 : Inport  Port=2  PortName=TCMSSystemInputs  Element=TractionSystem
  Bus Element In3 : Inport  Port=2  PortName=TCMSSystemInputs  Element=PneumaticsSystem
  In Bus Element6 : Inport  Port=2  PortName=TCMSSystemInputs  Element=PneumaticsSystem
  In Bus Element : Inport  Port=2  PortName=TCMSSystemInputs  Element=InputControlStates
  In Bus Element1 : Inport  Port=2  PortName=TCMSSystemInputs  Element=CBTC
  In Bus Element3 : Inport  Port=2  PortName=TCMSSystemInputs  Element=BrakingSystem
  In Bus Element8 : Inport  Port=2  PortName=TCMSSystemInputs  Element=DynamicsSystem
  Bus Element In4 : Inport  Port=3  PortName=WireStates  Element=TractionBrakingUnitSum
  In Bus Element2 : Inport  Port=3  PortName=WireStates  Element=TractionBrakingTrainWire
  In Bus Element4 : Inport  Port=3  PortName=WireStates  Element=TractionBrakingUnitWire
  In Bus Element5 : Inport  Port=3  PortName=WireStates  Element=PneumaticTrainSum
  In Bus Element7 : Inport  Port=4  PortName=Faults
  In Bus Element9 : Inport  Port=5  PortName=VehicleFaults
  Bus Creator : BusCreator  Inputs=2
  Goto Tag Visibility : GotoTagVisibility  GotoTag=EDBrakeRequested
  Goto Tag Visibility1 : GotoTagVisibility  GotoTag=SlipDetected
  Goto Tag Visibility2 : GotoTagVisibility  GotoTag=BECUFaulty
  Goto Tag Visibility3 : GotoTagVisibility  GotoTag=ASBogie1Deflated
  HoldingBrakeFB_ASDeflatedExtract : Subsystem
  TractionBrakingControl : Subsystem
  TractionBrakingDataExtract : Subsystem
  TractionBrakingDisplay : Subsystem
  TractionBrakingOut : Outport
  TractionBrakingUnitSumSources : Outport  Port=2
  TractionBrakingTrainWireSource : Outport  Port=3
  TractionBrakingUnitWireSources : Outport  Port=4
  tag scope: ASBogie1Deflated=scoped, EDBrakeRequested=scoped
  wires:
  TCMSSystemVehicleConfig/1 -> TractionBrakingDataExtract/1(TCMSSystemVehicleConfig), TractionBrakingDisplay/1(TCMSSystemVehicleConfig), TractionBrakingControl/1(TCMSConfig)
  Bus Element In2/1 -> TractionBrakingDisplay/12(TractionSystem), TractionBrakingControl/12(TractionSystem), TractionBrakingDataExtract/2(TractionSystem)
  Bus Element In1/1 -> TractionBrakingDisplay/3(ElectricalSignals), TractionBrakingControl/3(ElectricalSignals)
  Bus Element In/1 -> TractionBrakingDisplay/16(DisplayControl), TractionBrakingControl/4(DisplayControl)
  TractionBrakingDisplay/1(Display) -> Bus Creator/2
  TractionBrakingControl/2(Control) -> Bus Creator/1
  Bus Creator/1 -> TractionBrakingOut/1  "TractionBrakingOut"
  Bus Element In3/1 -> TractionBrakingDataExtract/3(PneumaticsSystem)
  TractionBrakingDataExtract/1(TractionBrakingVehicleData) -> TractionBrakingUnitSumSources/1, TractionBrakingDisplay/8(TractionVehicleData)
  TractionBrakingDataExtract/2(TractionBrakingBogieData) -> TractionBrakingControl/8(TractionBrakingBogieData), TractionBrakingDisplay/9(TractionOnBogieData)  "Bogie"
  Bus Element In4/1 -> TractionBrakingDisplay/5(TractionUnitData), TractionBrakingControl/6(TractionUnitData)
  In Bus Element/1 -> TractionBrakingDisplay/2(IOControl), TractionBrakingControl/2(InputControlStates)
  TractionBrakingControl/1(TractionBrakingTrainWireSource) -> TractionBrakingTrainWireSource/1
  In Bus Element1/1 -> TractionBrakingDisplay/7(CBTC), TractionBrakingControl/9(CBTCSignals)
  TractionBrakingControl/3(EDBrakeRequested) -> [EDBrakeRequested]
  In Bus Element3/1 -> TractionBrakingDisplay/13(BrakingSystem)
  TractionBrakingDataExtract/3(TractionBrakingUnitWireSources) -> TractionBrakingDisplay/10(TractionBrakingUnitData), TractionBrakingUnitWireSources/1
  In Bus Element4/1 -> TractionBrakingDisplay/11(TractionBrakingUW)
  In Bus Element5/1 -> TractionBrakingDisplay/6(PneumaticTrainSum), TractionBrakingControl/7(PneumaticTrainSum)
  In Bus Element7/1 -> TractionBrakingDisplay/14(Faults), TractionBrakingControl/11(Faults)
  In Bus Element6/1 -> HoldingBrakeFB_ASDeflatedExtract/2(PneumaticsIn), TractionBrakingControl/10(PneumaticsSystem)
  In Bus Element9/1 -> TractionBrakingControl/14(VehicleFaults), TractionBrakingDisplay/15(VehicleFaults)
  HoldingBrakeFB_ASDeflatedExtract/1(BusOut) -> TractionBrakingDisplay/4(TractionBrakingTW)
  In Bus Element2/1 -> HoldingBrakeFB_ASDeflatedExtract/1(WireStates), TractionBrakingControl/5(TractionTrainControl)
  HoldingBrakeFB_ASDeflatedExtract/2(ASBogie1Deflated) -> [ASBogie1Deflated]
  In Bus Element8/1 -> TractionBrakingControl/13(DynamicsSystem)

== system TCMSSystem/TCMSSystemPerVehicle/LimpHomeTCMSVehicle/CabUnitDisplay ==
  TCMSConfig : Inport
  ElectricalSignals : Inport  Port=2
  Bus Selector1 : BusSelector  OutputSignals=HasCab
  Bus Selector2 : BusSelector  OutputSignals=ElectricalSignals
  CabActiveUnitDisplay : Subsystem  TreatAsAtomicUnit=on
  Data Type Conversion : DataTypeConversion  OutDataTypeStr=uint32
  If : If  ShowElse=off
  CabUnitDisplay : Outport
  wires:
  CabActiveUnitDisplay/1(Out1) -> CabUnitDisplay/1
  If/1 -> CabActiveUnitDisplay/Action
  Data Type Conversion/1 -> If/1
  Bus Selector1/1 -> Data Type Conversion/1  "<HasCab>"
  TCMSConfig/1 -> Bus Selector1/1
  ElectricalSignals/1 -> Bus Selector2/1
  Bus Selector2/1 -> CabActiveUnitDisplay/1(ElectricalSignals)  "<ElectricalSignals>"

== system TCMSSystem/TCMSSystemPerVehicle/LimpHomeTCMSVehicle/TCMSTractionBraking ==
  note: This part of the model shall not be needed in
      | limp home mode except for the estimated mass.
      | Still retaining it for safety of the functionality.
  TCMSSystemVehicleConfig : Inport
  Bus Element In : Inport  Port=2  PortName=TCMSSystemInputs  Element=DisplayControl
  Bus Element In1 : Inport  Port=2  PortName=TCMSSystemInputs  Element=ElectricalSignals
  Bus Element In2 : Inport  Port=2  PortName=TCMSSystemInputs  Element=TractionSystem
  In Bus Element : Inport  Port=2  PortName=TCMSSystemInputs  Element=InputControlStates
  In Bus Element1 : Inport  Port=2  PortName=TCMSSystemInputs  Element=CBTC
  Bus Element In4 : Inport  Port=3  PortName=WireStates  Element=TractionBrakingUnitSum
  In Bus Element2 : Inport  Port=3  PortName=WireStates  Element=TractionBrakingTrainWire
  In Bus Element3 : Inport  Port=3  PortName=WireStates  Element=PneumaticTrainSum
  TractionBrakingControl : Subsystem
  TractionBrakingDataExtract : Subsystem
  TractionBrakingControls : Outport
  TractionBrakingUnitSumSources : Outport  Port=2
  TractionBrakingTrainWireSource : Outport  Port=3
  TractionBrakingUnitWireSources : Outport  Port=4
  wires:
  TCMSSystemVehicleConfig/1 -> TractionBrakingControl/1(TCMSConfig), TractionBrakingDataExtract/1(TCMSSystemVehicleConfig)
  Bus Element In2/1 -> TractionBrakingDataExtract/2(TractionSystem)
  Bus Element In1/1 -> TractionBrakingControl/3(ElectricalSignals)
  Bus Element In/1 -> TractionBrakingControl/4(DisplayControl)
  TractionBrakingControl/2(Control) -> TractionBrakingControls/1
  TractionBrakingDataExtract/1(TractionBrakingVehicleData) -> TractionBrakingUnitSumSources/1
  TractionBrakingDataExtract/2(TractionBrakingBogieData) -> TractionBrakingControl/8(TractionBrakingBogieData)  "Bogie"
  Bus Element In4/1 -> TractionBrakingControl/6(TractionUnitData)
  In Bus Element/1 -> TractionBrakingControl/2(InputControlStates)
  TractionBrakingControl/1(TractionBrakingTrainWireSource) -> TractionBrakingTrainWireSource/1
  In Bus Element2/1 -> TractionBrakingControl/5(TractionTrainControl)
  In Bus Element1/1 -> TractionBrakingControl/9(CBTCSignals)
  TractionBrakingDataExtract/3(TractionBrakingUnitWireSources) -> TractionBrakingUnitWireSources/1
  In Bus Element3/1 -> TractionBrakingControl/7(PneumaticTrainSum)

== system TCMSSystem/TCMSSystemPerVehicle/DisabledTCMSVehicle/CabUnitDisplay/CabActiveUnitDisplay ==
  Action Port : ActionPort  ActionPortLabel=if(u1 > 0)
  Bus Creator : BusCreator  Inputs=1
  Constant : Constant  Value=0
  Out1 : Outport
  wires:
  Bus Creator/1 -> Out1/1
  Constant/1 -> Bus Creator/1  "HMIPower"
